simulink subsystem "manipulability_and_collinearity"  (R2022b)
settings: Solver=VariableStepAuto  StartTime=0.0  StopTime=10.0  RelTol=1e-3
settings Model: Creator=emu  LastModifiedBy=emu

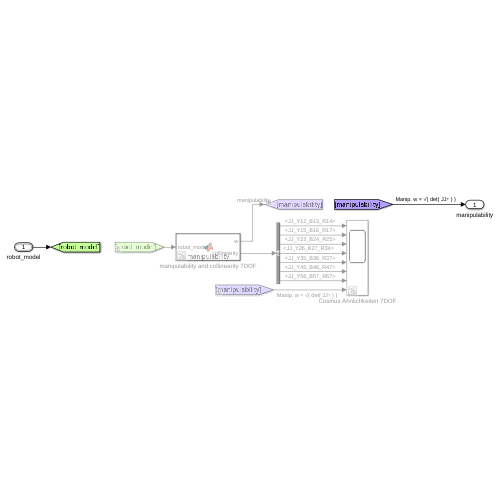
[thumbnail: Simulink's stored preview of the top-level diagram]
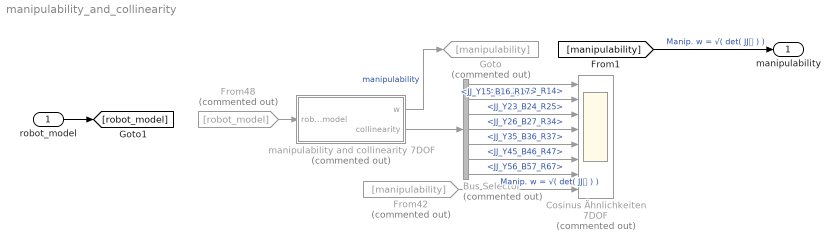
== system manipulability_and_collinearity ==
  robot_model : Inport  OutDataTypeStr=Bus: robot_model
  Bus Selector : BusSelector  Commented=on  OutputSignals=JJ_Y12_B13_R14,JJ_Y15_B16_R17,JJ_Y23_B24_R25,JJ_Y26_B27_R34,JJ_Y35_B36_R37,JJ_Y45_B46_R47,JJ_Y56_B57_R67
  Cosinus Ähnlichkeiten 7DOF : Scope  Commented=on  NumInputPorts=8
  From42 : From  Commented=on  GotoTag=manipulability
  From48 : From  Commented=on  GotoTag=robot_model
  Goto : Goto  Commented=on  GotoTag=manipulability
  manipulability and collinearity 7DOF : MATLAB Function  Commented=on  TreatAsAtomicUnit=on
  manipulability : Outport
  wires:
  manipulability and collinearity 7DOF/1(w) -> Goto/1  "manipulability"
  Bus Selector/6 -> Cosinus Ähnlichkeiten 7DOF/6  "<JJ_Y45_B46_R47>"
  Bus Selector/3 -> Cosinus Ähnlichkeiten 7DOF/3  "<JJ_Y23_B24_R25>"
  From48/1 -> manipulability and collinearity 7DOF/1(robot_model)
  Bus Selector/4 -> Cosinus Ähnlichkeiten 7DOF/4  "<JJ_Y26_B27_R34>"
  Bus Selector/5 -> Cosinus Ähnlichkeiten 7DOF/5  "<JJ_Y35_B36_R37>"
  Bus Selector/1 -> Cosinus Ähnlichkeiten 7DOF/1  "<JJ_Y12_B13_R14>"
  Bus Selector/7 -> Cosinus Ähnlichkeiten 7DOF/7  "<JJ_Y56_B57_R67>"
  From42/1 -> Cosinus Ähnlichkeiten 7DOF/8  "Manip. w = √( det( JJ⸆ ) )"
  manipulability and collinearity 7DOF/2(collinearity) -> Bus Selector/1
  Bus Selector/2 -> Cosinus Ähnlichkeiten 7DOF/2  "<JJ_Y15_B16_R17>"
  robot_model/1 -> [robot_model]
  [manipulability] -> manipulability/1  "Manip. w = √( det( JJ⸆ ) )"

== matlab function manipulability_and_collinearity/manipulability and collinearity 7DOF ==
  settings: sampleTime=param_global.Ta
  data: robot_model input; w output; init_bus_param parameter; collinearity output Bus: collinearity_bus
function [w, collinearity]   = manipulability(robot_model, init_bus_param)

J = robot_model.J;
det_J = det(J*J');
w = sqrt(abs(det_J));

J_tilde = J./vecnorm(J);
JJ_colin = J_tilde'*J_tilde;

collinearity = init_bus_param.init_collinearity_bus;

% 7DOF
collinearity.JJ_Y12_B13_R14 = [JJ_colin(1,2); JJ_colin(1,3); JJ_colin(1,4)];
collinearity.JJ_Y15_B16_R17 = [JJ_colin(1,5); JJ_colin(1,6); JJ_colin(1,7)];
collinearity.JJ_Y23_B24_R25 = [JJ_colin(2,3); JJ_colin(2,4); JJ_colin(2,5)];
collinearity.JJ_Y26_B27_R34 = [JJ_colin(2,6); JJ_colin(2,7); JJ_colin(3,4)];
collinearity.JJ_Y35_B36_R37 = [JJ_colin(3,5); JJ_colin(3,6); JJ_colin(3,7)];
collinearity.JJ_Y45_B46_R47 = [JJ_colin(4,5); JJ_colin(4,6); JJ_colin(4,7)];
collinearity.JJ_Y56_B57_R67 = [JJ_colin(5,6); JJ_colin(5,7); JJ_colin(6,7)];
